simulink model "A02_L3_1esantionare"  (R2014b)
settings: Solver=ode3  StartTime=0.0  StopTime=5  FixedStep=1e-5  RelTol=1e-3
values from neighbouring files (symbols this model uses):
  C1 = 220*(0.1+b)*10^(-6)    (= 2.2e-05)    [A03_L3_1script.m]
  C2 = C1+(a+5)*10^(-6)    (= 2.7e-05)    [A03_L3_1script.m]
  R1 = 120*(0.1+b)+10*(a+1)    (= 22)    [A03_L3_1script.m]
  R2 = 430-15*(a+2)    (= 400)    [A03_L3_1script.m]
libraries: simulink x2
settings Model: Creator=User  LastModifiedBy=User

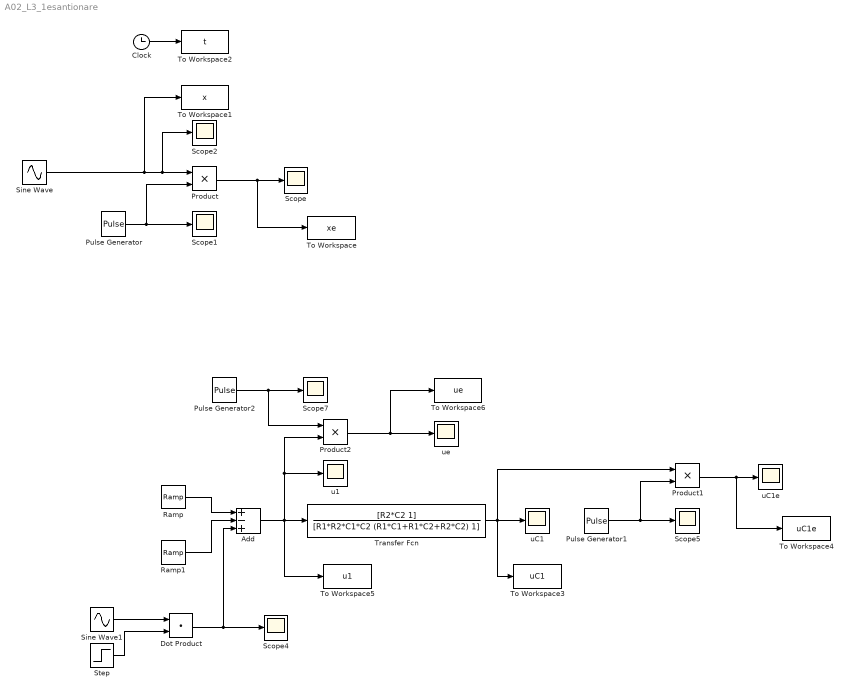
== system A02_L3_1esantionare ==
  Add : Sum  Inputs=+-+
  Clock : Clock
  Dot Product : DotProduct  InputSameDT=on  OutDataTypeStr=Inherit: Inherit via internal rule
  Product : Product
  Product1 : Product
  Product2 : Product
  Pulse Generator : DiscretePulseGenerator  PulseType=Time based  Period=0.2  PulseWidth=0.1
  Pulse Generator1 : DiscretePulseGenerator  PulseType=Time based  Period=0.33  PulseWidth=0.1
  Pulse Generator2 : DiscretePulseGenerator  PulseType=Time based  Period=0.26  PulseWidth=0.1
  Ramp : simulink/Sources/Ramp  slope=12.5  start=1  X0=0
  Ramp1 : simulink/Sources/Ramp  slope=12.5  start=4  X0=0
  Scope{,1..2,4..5,7} (6 alike) : Scope
      Scope settings: TimeRange=5  YMin=0  YMax=3  MaxDataPoints=500000
      Scope1 settings: MaxDataPoints=500000
      Scope2 settings: SaveName=ScopeData2  MaxDataPoints=500000
      Scope4 settings: SaveName=ScopeData4  MaxDataPoints=50000
      Scope5 settings: SaveName=ScopeData7  MaxDataPoints=50000
      Scope7 settings: SaveName=ScopeData9  MaxDataPoints=50000
  Sine Wave : Sin  Amplitude=3.5  Frequency=2*pi  Phase=0.16  SampleTime=0
  Sine Wave1 : Sin  Amplitude=3  Frequency=200  SampleTime=0
  Step : Step  SampleTime=0
  To Workspace : ToWorkspace  VariableName=xe  SampleTime=-1
  To Workspace1 : ToWorkspace  VariableName=x  SampleTime=-1
  To Workspace2 : ToWorkspace  VariableName=t  SampleTime=-1
  To Workspace3 : ToWorkspace  VariableName=uC1  SampleTime=-1
  To Workspace4 : ToWorkspace  VariableName=uC1e  SampleTime=-1
  To Workspace5 : ToWorkspace  VariableName=u1  SampleTime=-1
  To Workspace6 : ToWorkspace  VariableName=ue  SampleTime=-1
  Transfer Fcn : TransferFcn  Numerator=[R2*C2 1]  Denominator=[R1*R2*C1*C2 (R1*C1+R1*C2+R2*C2) 1]
  u1 : Scope
      settings: SaveName=ScopeData5  MaxDataPoints=50000
  uC1 : Scope
      settings: YMin=-1  YMax=1  SaveName=ScopeData6  MaxDataPoints=50000
  uC1e : Scope
      settings: SaveName=ScopeData8  MaxDataPoints=500000
  ue : Scope
      settings: YMin=0  YMax=25  SaveName=ScopeData10  MaxDataPoints=500000
  wires:
  Clock/1 -> To Workspace2/1
  Sine Wave/1 -> To Workspace1/1, Scope2/1, Product/1
  Product/1 -> To Workspace/1, Scope/1
  Pulse Generator/1 -> Product/2, Scope1/1
  Add/1 -> To Workspace5/1, Product2/2, u1/1, Transfer Fcn/1
  Ramp/1 -> Add/1
  Ramp1/1 -> Add/2
  Sine Wave1/1 -> Dot Product/1
  Step/1 -> Dot Product/2
  Dot Product/1 -> Scope4/1, Add/3
  Transfer Fcn/1 -> Product1/1, To Workspace3/1, uC1/1
  Product1/1 -> To Workspace4/1, uC1e/1
  Pulse Generator1/1 -> Product1/2, Scope5/1
  Product2/1 -> To Workspace6/1, ue/1
  Pulse Generator2/1 -> Product2/1, Scope7/1
